simulink model "Simulator_Case_9"  (R2024a)
settings: Solver=VariableStepAuto  StartTime=0.0  StopTime=1400  RelTol=1e-3
values from neighbouring files (symbols this model uses):
  Declination_Sigean = 2.116*(pi/180)    (= 0.0369311669722)    [Parametrization_Simulation_Case_9.m]
  Position_Initial_X = Waypoints_X(1)    [Parametrization_Simulation_Case_9.m]
  Position_Initial_Y = Waypoints_Y(1)    [Parametrization_Simulation_Case_9.m]
  Time_Period_Sampling = 0.1    [Parametrization_Simulation_Case_9.m]
  Velocity_Norm_Ship_Initial = 6/3.6    (= 1.66666666667)    [Parametrization_Simulation_Case_9.m]
undefined symbols (not defined in the file or in its folder): Damping_Coefficient, Damping_Factor_Waves, Density_Water_Salted, Draft_Depth, Drag_Coefficient, Gain_Filter, Inertia_Moment, Length_Ship, Longeron_Area, Mass_Ship, Pulsation_Natural, Pulsation_Wave, Rudder_Angle_Maximal, Rudder_Angle_Minimal, Rudder_Rate_Maximal, Rudder_Rate_Minimal, Static_Gain_Nomoto, Time_Constant_Total, Waypoints
libraries: cstblocks x2, simulink_extras x1
(part 2 of 2)

== matlab function Simulator_Case_9/Dynamics_Kinematics_Ship_Propagation/Dynamics_Ship_Heading_Rudder/Ship_LPV_Velocity ==
  data: Velocity_Current input; Static_Gain_Nomoto output; Length_Ship_Current input; Density_Water_Current input; Drag_Coefficient_Current input; Draft_Depth_Current input; Longeron_Area_Current input; Mass_Of_The_Ship_Current input; Time_Constant_Total output; Static_Gain_Over_Time output; Inverse_Time output; Velocity_Initial input; Time_Constant_1_Plus_2_Over_1_Times_2 output; Gain_Sway_Times_Time_Sway_Over_Times_Products output; Ineverse_Time_1_Times_2 output; Gain_Sway_Over_Product_Times output
function [Static_Gain_Nomoto,...
          Time_Constant_Total,...
          Static_Gain_Over_Time,...
          Inverse_Time,...
          Time_Constant_1_Plus_2_Over_1_Times_2,...
          Gain_Sway_Times_Time_Sway_Over_Times_Products,...
          Ineverse_Time_1_Times_2,...
          Gain_Sway_Over_Product_Times] = Static_Gain_Time_Constant_Varying_Velocity(Velocity_Current,...
                                                                                     Length_Ship_Current,...
                                                                                     Density_Water_Current,...
                                                                                     Drag_Coefficient_Current,...
                                                                                     Draft_Depth_Current,...
                                                                                     Longeron_Area_Current,...
                                                                                     Mass_Of_The_Ship_Current,...
                                                                                     Velocity_Initial)


% Only the velocity will be taken into account at first, but all the other terms
% and parameters are considered in inputs for future potential dispersions
% considerations.

% Protection for null velocity declaration:
if Velocity_Current == 0
    Velocity_Current = Velocity_Initial;
end

% Call of the embedded estimation function:
[Static_Gain_Nomoto,...
 Time_Constant_Total,...
 Time_Constant_1,...
 Time_Constant_2,...
 Time_Constant_3,...
 Time_Constant_Sway,...
 Static_Gain_Sway] = Static_Gain_Time_Constant_Varying_Velocity_Embedded(Velocity_Current,...
                                                                         Length_Ship_Current,...
                                                                         Density_Water_Current,...
                                                                         Drag_Coefficient_Current,...
                                                                         Draft_Depth_Current,...
                                                                         Longeron_Area_Current,...
                                                                         Mass_Of_The_Ship_Current);

% Final operations for LPV Function:
Static_Gain_Over_Time = Static_Gain_Nomoto/Time_Constant_Total;
Inverse_Time = 1/Time_Constant_Total;
Time_Constant_1_Plus_2_Over_1_Times_2 = (Time_Constant_1 + Time_Constant_2)/(Time_Constant_1*Time_Constant_2);
Ineverse_Time_1_Times_2 = 1/(Time_Constant_1*Time_Constant_2);
Gain_Sway_Times_Time_Sway_Over_Times_Products = (Static_Gain_Sway*Time_Constant_Sway)/(Time_Constant_1*Time_Constant_2);
Gain_Sway_Over_Product_Times = Static_Gain_Sway/(Time_Constant_1*Time_Constant_2);

end

== matlab function Simulator_Case_9/Guidance_Integration_Line_Of_Sight/Guidance_Algorithm ==
  settings: updateMethod=DISCRETE
  data: Heading_Reference_Aimed_Raw output; Waypoints input; Position_X_Ship_Current input; Position_Y_Ship_Current input; Cross_Track_Error_Current output; Time_Sampling input; Position_X_Ship_Initial input; Position_Y_Ship_Initial input; Time_Current input
function [Heading_Reference_Aimed_Raw,...
          Cross_Track_Error_Current] = Guidance_Integration_Line_Of_Sight(Waypoints,...
                                                                          Position_X_Ship_Current,...
                                                                          Position_Y_Ship_Current,...
                                                                          Time_Sampling,...
                                                                          Position_X_Ship_Initial,...
                                                                          Position_Y_Ship_Initial,...
                                                                          Time_Current)


% The Guidance function is based on a PI scheme integrated to the embedded
% algorithm. It is of the Line-Of-Sight (LOS) type.
[Heading_Reference_Aimed_Raw,...
 Cross_Track_Error_Current] = Guidance_Integrated_Line_Of_Sight(Waypoints,...
                                                                Position_X_Ship_Current,...
                                                                Position_Y_Ship_Current,...
                                                                Time_Sampling,...
                                                                Position_X_Ship_Initial,...
                                                                Position_Y_Ship_Initial,...
                                                                Time_Current);

end

== matlab function Simulator_Case_9/Controller_Actuator/Controller/H_Infinity_Controller_Synthetized ==
  data: Heading_Aimed_Current input; Rudder_Angle_Elaborated_Current output; Heading_Observed_Current input; Time_Sampling input
function Rudder_Angle_Elaborated_Current = Synthetized_Controller_H_Infinity(Heading_Aimed_Current,...
                                                                             Heading_Observed_Current,...
                                                                             Time_Sampling)

% Controller obtained via H_Infinity Standard Stochastic Optimization. The
% final controller has been chosen to be of order 3:
Rudder_Angle_Elaborated_Current = Controller_Optimal_H_Infinity_Synthesis(Heading_Aimed_Current,...
                                                                          Heading_Observed_Current,...
                                                                          Time_Sampling);

end

== matlab function Simulator_Case_9/Guidance_Integration_Line_Of_Sight/Guidance_Reference_Model ==
  data: Heading_Raw_Aimed input; Heading_Desired_Current output; Time_Sampling input; Angular_Rate_Desired_Current output; Angular_Acceleration_Desired_Current output
function [Heading_Desired_Current,...
          Angular_Rate_Desired_Current,...
          Angular_Acceleration_Desired_Current] = Guidance_Model_Reference_To_Desired(Heading_Raw_Aimed,...
                                                                                      Time_Sampling)

% Reference model used to make more realistic profiles Guidance in terms of
% aimed Heading angle, incorporating limitations of the rudder actuators.
[Heading_Desired_Current,...
 Angular_Rate_Desired_Current,...
 Angular_Acceleration_Desired_Current] = Guidance_Model_Reference(Heading_Raw_Aimed,...
                                                                  Time_Sampling);

end
